simulink model "simulink_mecha_discrete_TEST"  (R2016b)
settings: Solver=ode1  StartTime=0.0  StopTime=10  FixedStep=0.01  RelTol=1e-6
undefined symbols (not defined in the file or in its folder): DiscIntNeverNeededParam
libraries: simulink x2, dspinverses x1
settings Model: Creator=Utente  LastModifiedBy=liana
settings DataIOCC: SaveState=on
settings OptimizationCC: BlockReduction=off  DefaultParameterBehavior=Inlined  BufferReuse=off

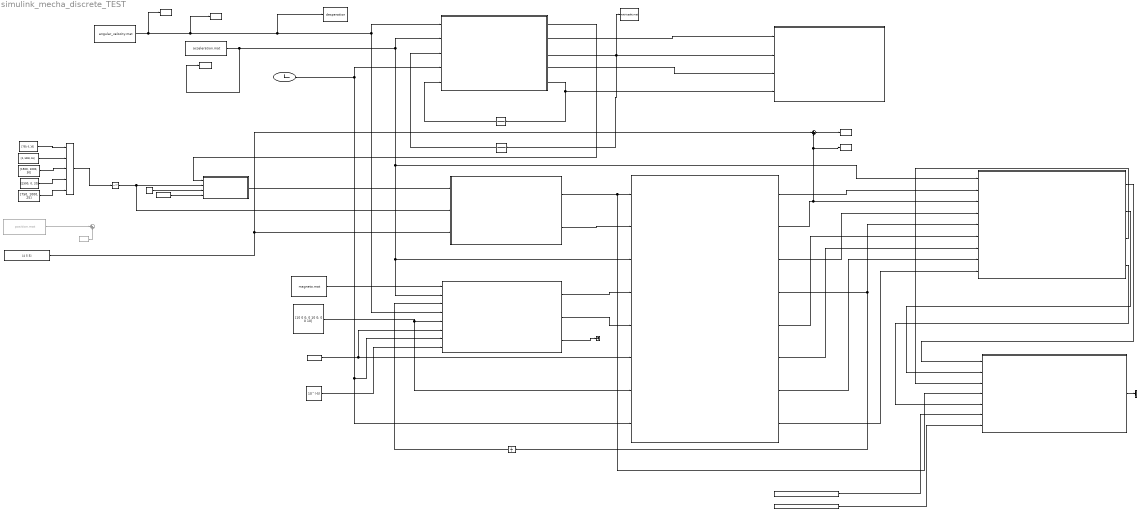
== system simulink_mecha_discrete_TEST ==
  Attitude Observer : Subsystem
  Band-Limited White Noise1 : simulink/Sources/Band-Limited White Noise  Commented=on  Cov=[0.1; 0.1; 0.1]  Ts=0.1  seed=[23341]
  Clock : Clock
      settings: Decimation=50
  Discrete-Time Integrator : DiscreteIntegrator  IntegratorMethod=Integration: Trapezoidal  InitialConditionSetting=State (most efficient)  SampleTime=-1  ICPrevOutput=DiscIntNeverNeededParam  ICPrevScaledInput=DiscIntNeverNeededParam
  Discrete-Time Integrator1 : DiscreteIntegrator  IntegratorMethod=Integration: Trapezoidal  InitialConditionSetting=State (most efficient)  SampleTime=-1  ICPrevOutput=DiscIntNeverNeededParam  ICPrevScaledInput=DiscIntNeverNeededParam
  Displays : Subsystem
  From  p_n_vehicle : FromFile  Commented=on  FileName=position.mat  SampleTime=0
  From acceleration file : FromFile  FileName=acceleration.mat  SampleTime=0
  From angular_velocity file : FromFile  FileName=angular_velocity.mat  SampleTime=0
  From magnetometer file : FromFile  FileName=magneto.mat  SampleTime=0  InterpolationWithinTimeRange=Zero order hold
  Kalman - Bucy Filter : Subsystem
  Kp : Constant  Value=[10 0 0; 0 10 0; 0 0 10]
  Local linearization1 : Subsystem
  Math Function : Math  Operator=transpose  SaturateOnIntegerOverflow=on
  Matrix Concatenate : Concatenate  NumInputs=5  Mode=Multidimensional array  ConcatenateDimension=2
  Mechanisation subsystem : Subsystem
  Nonlinear algebraic transform and solution : Subsystem
  Q matrix : Constant  Value=diag([0, 0, 0, 10^-5, 10^-3, 10^-3, 10^-3, 10^-8, 10^-8, 10^-8])
  R matrix : Constant  Value=0.25*diag([1 1 1 1])
  Sum : Sum  Inputs=|++
  Sum1 : Sum  Commented=on  Inputs=|++
  Terminator : Terminator
  Terminator2 : Terminator
  To File : ToFile  Filename=matricedot.mat  MatrixName=md  SaveFormat=Timeseries
  To Workspace : ToWorkspace  VariableName=desperation  SampleTime=-1
  To Workspace1 : ToWorkspace  VariableName=ang_vel  SampleTime=-1
  To Workspace2 : ToWorkspace  VariableName=ang_vel_dist  SampleTime=-1
  To Workspace3 : ToWorkspace  VariableName=accel  SaveFormat=Timeseries  SampleTime=-1
  To Workspace4 : ToWorkspace  VariableName=p_n  SaveFormat=Timeseries  SampleTime=-1
  To Workspace5 : ToWorkspace  VariableName=p_n_delta_stim  SaveFormat=Timeseries  SampleTime=-1
  Translational Motion Observer : Subsystem
  Unit Delay : UnitDelay  SampleTime=-1
  beta : Constant
  epsilon : Constant  Value=[1 1 1 1 1]
  ki : Constant  Value=10^(-5)
  p_n_1 : Constant  Value=[750, 0, 10]
  p_n_2 : Constant  Value=[0, 1000, 15]
  p_n_3 : Constant  Value=[1500, 1000, 30]
  p_n_4 : Constant  Value=[1500, 0, 20]
  p_n_5 : Constant  Value=[750, 1000, 25]
  position_0_fixed_reference : Constant  Value=[4 5 5]
  pseudorange_measurement_model : MATLAB Function  TreatAsAtomicUnit=on
  sigma : Constant  Value=0.25
  wires:
  Clock/1 -> Attitude Observer/7(t), Translational Motion Observer/8(t), Mechanisation subsystem/4(t)
  Mechanisation subsystem/3(R_nb_dot) -> Discrete-Time Integrator1/1, To File/1, Displays/2(R_nb_dot)
  Mechanisation subsystem/2(v_n_dot) -> Displays/1(v_n_dot)
  Mechanisation subsystem/4(v_n_dot_noise) -> Displays/3(v_n_dot_noise)
  Mechanisation subsystem/5(R_nb_dot_noise) -> Discrete-Time Integrator/1, Displays/4(R_nb_dot_noise)
  Discrete-Time Integrator/1 -> Mechanisation subsystem/5(R_nb_noise)
  Discrete-Time Integrator1/1 -> Mechanisation subsystem/3(R_nb)
  Nonlinear algebraic transform and solution/1(delta) -> Kalman - Bucy Filter/4(sensors measurements), Translational Motion Observer/1(delta)
  Translational Motion Observer/4(f_n_stim) -> Local linearization1/5(f_n_stim), Unit Delay/1
  Attitude Observer/1(J) -> Translational Motion Observer/4(J)
  Attitude Observer/2(R_nb_stim) -> Translational Motion Observer/5(R_nb_stim)
  Attitude Observer/3(b_stim) -> Terminator/1
  Kp/1 -> Translational Motion Observer/7(Kp), Attitude Observer/5(Kp)
  sigma/1 -> Attitude Observer/6(sigma), Translational Motion Observer/6(sigma)
  Translational Motion Observer/3(v_n_stim) -> Local linearization1/4(v_n_stim)
  Nonlinear algebraic transform and solution/2(C_dx) -> Translational Motion Observer/2(C_dx)
  Local linearization1/1(AL) -> Kalman - Bucy Filter/1(AL)
  Local linearization1/2(BL) -> Kalman - Bucy Filter/2(BL)
  Local linearization1/3(CL) -> Kalman - Bucy Filter/3(CL)
  pseudorange_measurement_model/1(y) -> Nonlinear algebraic transform and solution/1(y)
  Local linearization1/4(U) -> Kalman - Bucy Filter/5(U)
  beta/1 -> pseudorange_measurement_model/3(beta)
  epsilon/1 -> pseudorange_measurement_model/4(epsilon)
  Matrix Concatenate/1 -> Math Function/1
  R matrix/1 -> Kalman - Bucy Filter/6(R)
  Q matrix/1 -> Kalman - Bucy Filter/7(Q)
  Kalman - Bucy Filter/1(Out1) -> Terminator2/1
  Translational Motion Observer/5(K) -> Local linearization1/6(K)
  Translational Motion Observer/6("C ") -> Local linearization1/7(C)
  Translational Motion Observer/7(" A") -> Local linearization1/8(A)
  Translational Motion Observer/8(B) -> Local linearization1/9(B)
  ki/1 -> Attitude Observer/8(Ki)
  Unit Delay/1 -> Attitude Observer/3(f_n_stim)
  Band-Limited White Noise1/1 -> Sum1/2
  From  p_n_vehicle/1 -> Sum1/1
  Translational Motion Observer/1(beta_stim) -> Local linearization1/2(beta_stim)
  Translational Motion Observer/2(p_n_delta_stim) -> To Workspace5/1, Sum/2, Local linearization1/3(p_n_stim)
  Mechanisation subsystem/1(p_n) -> pseudorange_measurement_model/1(p_n)
  p_n_5/1 -> Matrix Concatenate/5
  p_n_4/1 -> Matrix Concatenate/4
  p_n_3/1 -> Matrix Concatenate/3
  p_n_2/1 -> Matrix Concatenate/2
  p_n_1/1 -> Matrix Concatenate/1
  Math Function/1 -> Nonlinear algebraic transform and solution/2(p), pseudorange_measurement_model/2(p_n_i)
  From angular_velocity file/1 -> To Workspace/1, Attitude Observer/4(w_ib), Mechanisation subsystem/1(w_ib), To Workspace2/1, To Workspace1/1
  From acceleration file/1 -> Local linearization1/1(f_b_imu), Attitude Observer/2(f_b), Translational Motion Observer/3(f_b_imu), Mechanisation subsystem/2(f_b), To Workspace3/1
  From magnetometer file/1 -> Attitude Observer/1(m_b_mag)
  Sum/1 -> To Workspace4/1
  position_0_fixed_reference/1 -> Sum/1, Nonlinear algebraic transform and solution/3(p0)

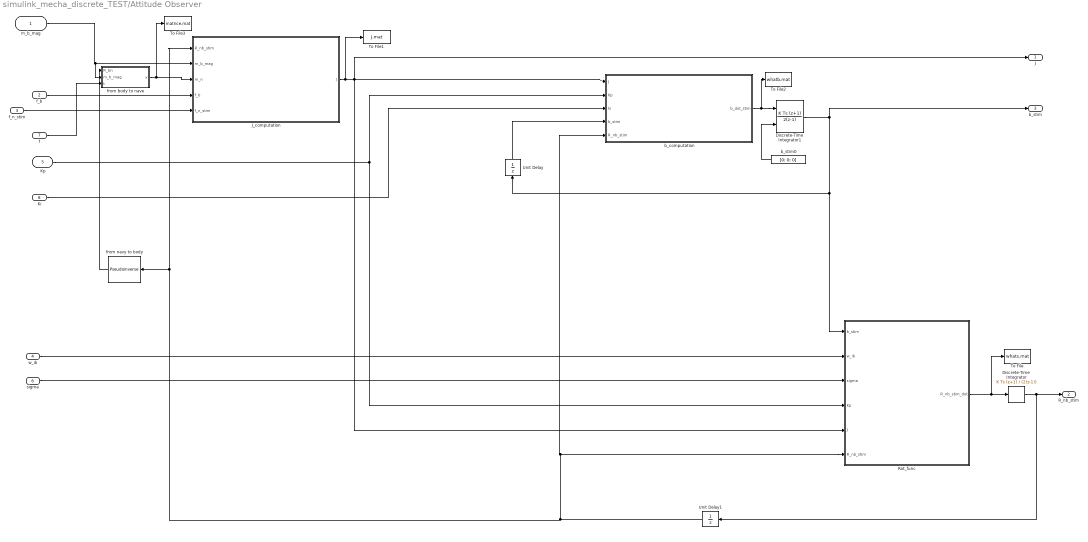
== system simulink_mecha_discrete_TEST/Attitude Observer ==
  m_b_mag : Inport
  f_b : Inport  Port=2
  f_n_stim : Inport  Port=3
  w_ib : Inport  Port=4
  Kp : Inport  Port=5
  sigma : Inport  Port=6
  t : Inport  Port=7
  Ki : Inport  Port=8
  Discrete-Time Integrator : DiscreteIntegrator  IntegratorMethod=Integration: Trapezoidal  InitialConditionSetting=State (most efficient)  SampleTime=-1  ICPrevOutput=DiscIntNeverNeededParam  ICPrevScaledInput=DiscIntNeverNeededParam
  Discrete-Time Integrator1 : DiscreteIntegrator  IntegratorMethod=Integration: Trapezoidal  InitialConditionSource=external  InitialConditionSetting=State (most efficient)  SampleTime=-1  ICPrevOutput=DiscIntNeverNeededParam  ICPrevScaledInput=DiscIntNeverNeededParam
  J_computation : Subsystem
  Rot_func : MATLAB Function  TreatAsAtomicUnit=on
  To File : ToFile  Filename=whats.mat  SaveFormat=Timeseries
  To File1 : ToFile  Filename=J.mat  MatrixName=J  SaveFormat=Timeseries
  To File2 : ToFile  Filename=whatb.mat  MatrixName=b  SaveFormat=Timeseries
  To File3 : ToFile  Filename=matrice.mat  MatrixName=m  SaveFormat=Timeseries
  Unit Delay : UnitDelay  SampleTime=-1
  Unit Delay1 : UnitDelay  SampleTime=-1
  b_computation : MATLAB Function  TreatAsAtomicUnit=on
  b_stim0 : Constant  Value=[0; 0; 0]
  from body to nave : MATLAB Function  TreatAsAtomicUnit=on
  from navy to body : dspinverses/Pseudoinverse  wanterr=off  SimulateUsing=Interpreted execution
  J : Outport
  R_nb_stim : Outport  Port=2
  b_stim : Outport  Port=3
  wires:
  m_b_mag/1 -> from body to nave/2(m_b_mag), J_computation/2(m_b_mag)
  Rot_func/1(R_nb_stim_dot) -> Discrete-Time Integrator/1, To File/1
  b_computation/1(b_dot_stim) -> Discrete-Time Integrator1/1, To File2/1
  Discrete-Time Integrator1/1 -> b_stim/1, Unit Delay/1, Rot_func/1(b_stim)
  from body to nave/1(y) -> J_computation/3(m_n), To File3/1
  f_b/1 -> J_computation/4(f_b)
  f_n_stim/1 -> J_computation/5(f_n_stim)
  J_computation/1(J) -> To File1/1, J/1, Rot_func/5(J), b_computation/1(J)
  Kp/1 -> b_computation/2(Kp), Rot_func/4(Kp)
  Ki/1 -> b_computation/3(ki)
  sigma/1 -> Rot_func/3(sigma)
  w_ib/1 -> Rot_func/2(w_ib)
  t/1 -> from body to nave/3(t)
  Discrete-Time Integrator/1 -> R_nb_stim/1, Unit Delay1/1
  Unit Delay/1 -> b_computation/4(b_stim)
  Unit Delay1/1 -> from navy to body/1, J_computation/1(R_nb_stim), b_computation/5(R_nb_stim), Rot_func/6(R_nb_stim)
  from navy to body/1 -> from body to nave/1(R_bn)
  b_stim0/1 -> Discrete-Time Integrator1/2

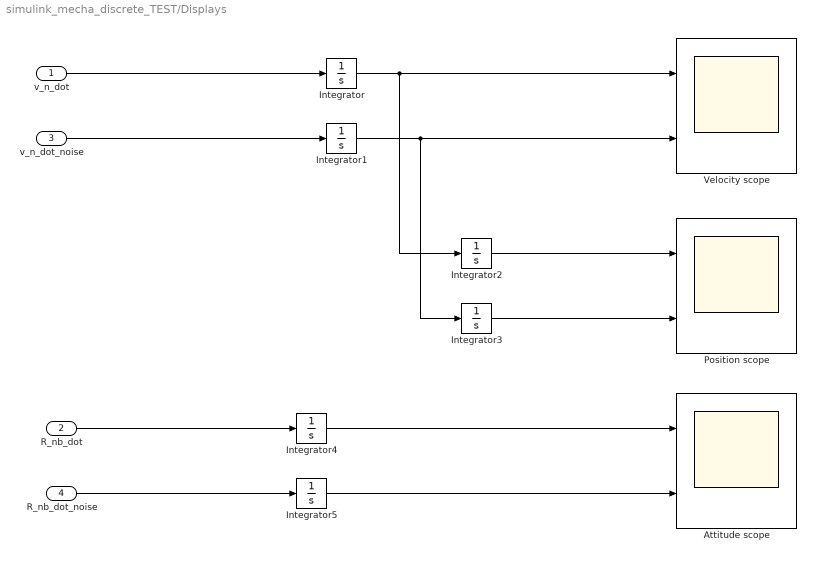
== system simulink_mecha_discrete_TEST/Displays ==
  v_n_dot : Inport
  R_nb_dot : Inport  Port=2
  v_n_dot_noise : Inport  Port=3
  R_nb_dot_noise : Inport  Port=4
  Attitude scope : Scope  NumInputPorts=2
  Integrator{,1..5} (6 alike) : Integrator
  Position scope : Scope  NumInputPorts=2
  Velocity scope : Scope  NumInputPorts=2
  wires:
  v_n_dot/1 -> Integrator/1
  v_n_dot_noise/1 -> Integrator1/1
  Integrator/1 -> Integrator2/1, Velocity scope/1
  Integrator1/1 -> Integrator3/1, Velocity scope/2
  Integrator2/1 -> Position scope/1
  Integrator3/1 -> Position scope/2
  R_nb_dot/1 -> Integrator4/1
  R_nb_dot_noise/1 -> Integrator5/1
  Integrator4/1 -> Attitude scope/1
  Integrator5/1 -> Attitude scope/2

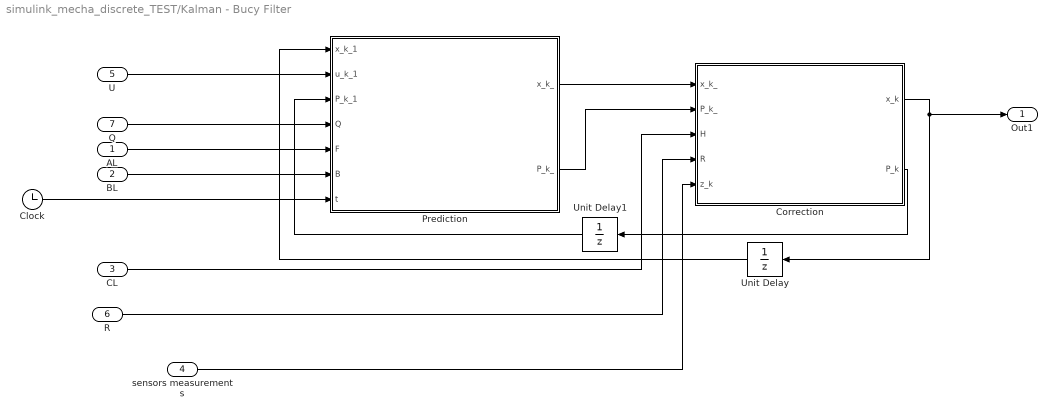
== system simulink_mecha_discrete_TEST/Kalman - Bucy Filter ==
  AL : Inport
  BL : Inport  Port=2
  CL : Inport  Port=3
  sensors measurements : Inport  Port=4
  U : Inport  Port=5
  R : Inport  Port=6
  Q : Inport  Port=7
  Clock : Clock
  Correction : MATLAB Function  TreatAsAtomicUnit=on
  Prediction : MATLAB Function  TreatAsAtomicUnit=on
  Unit Delay : UnitDelay  SampleTime=-1
  Unit Delay1 : UnitDelay  SampleTime=-1
  Out1 : Outport
  wires:
  Prediction/2(P_k_) -> Correction/2(P_k_)
  Prediction/1(x_k_) -> Correction/1(x_k_)
  Correction/2(P_k) -> Unit Delay1/1
  Correction/1(x_k) -> Unit Delay/1, Out1/1
  AL/1 -> Prediction/5(F)
  CL/1 -> Correction/3(H)
  Clock/1 -> Prediction/7(t)
  Q/1 -> Prediction/4(Q)
  sensors measurements/1 -> Correction/5(z_k)
  BL/1 -> Prediction/6(B)
  U/1 -> Prediction/2(u_k_1)
  R/1 -> Correction/4(R)
  Unit Delay/1 -> Prediction/1(x_k_1)
  Unit Delay1/1 -> Prediction/3(P_k_1)

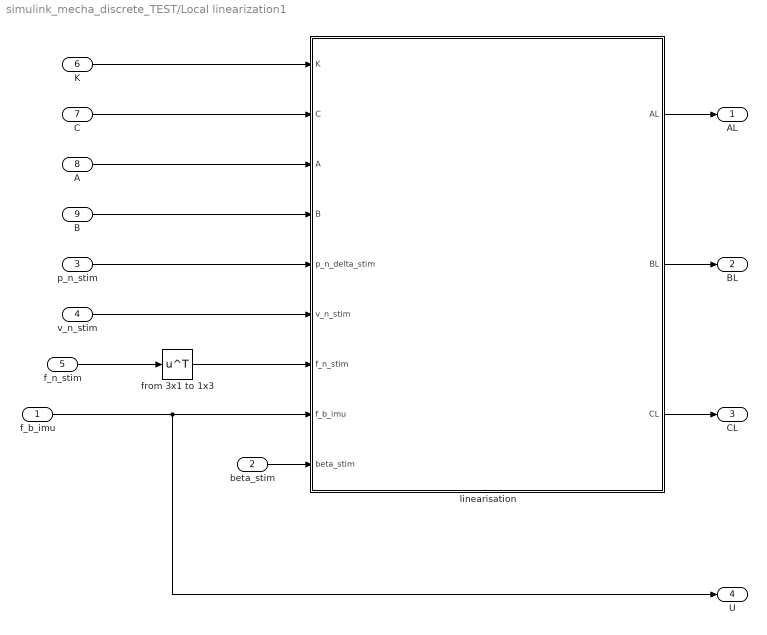
== system simulink_mecha_discrete_TEST/Local linearization1 ==
  f_b_imu : Inport
  beta_stim : Inport  Port=2
  p_n_stim : Inport  Port=3
  v_n_stim : Inport  Port=4
  f_n_stim : Inport  Port=5
  K : Inport  Port=6
  C : Inport  Port=7
  A : Inport  Port=8
  B : Inport  Port=9
  from 3x1 to 1x3 : Math  Operator=transpose  SaturateOnIntegerOverflow=on
  linearisation : MATLAB Function  TreatAsAtomicUnit=on
  AL : Outport
  BL : Outport  Port=2
  CL : Outport  Port=3
  U : Outport  Port=4
  wires:
  linearisation/1(AL) -> AL/1
  linearisation/2(BL) -> BL/1
  linearisation/3(CL) -> CL/1
  K/1 -> linearisation/1(K)
  C/1 -> linearisation/2(C)
  A/1 -> linearisation/3(A)
  B/1 -> linearisation/4(B)
  p_n_stim/1 -> linearisation/5(p_n_delta_stim)
  beta_stim/1 -> linearisation/9(beta_stim)
  f_n_stim/1 -> from 3x1 to 1x3/1
  v_n_stim/1 -> linearisation/6(v_n_stim)
  f_b_imu/1 -> U/1, linearisation/8(f_b_imu)
  from 3x1 to 1x3/1 -> linearisation/7(f_n_stim)

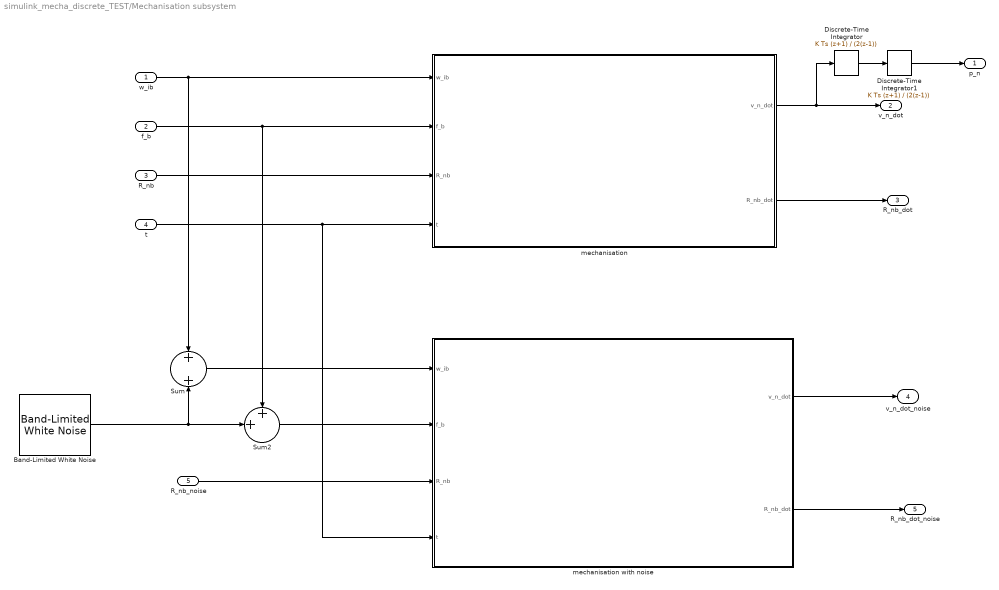
== system simulink_mecha_discrete_TEST/Mechanisation subsystem ==
  w_ib : Inport
  f_b : Inport  Port=2
  R_nb : Inport  Port=3
  t : Inport  Port=4
  R_nb_noise : Inport  Port=5
  Band-Limited White Noise : simulink/Sources/Band-Limited White Noise  Cov=[100 100 100]'  Ts=0.1  seed=[23341]  VectorParams1D=off
  Discrete-Time Integrator : DiscreteIntegrator  IntegratorMethod=Integration: Trapezoidal  InitialConditionSetting=State (most efficient)  SampleTime=-1  ICPrevOutput=DiscIntNeverNeededParam  ICPrevScaledInput=DiscIntNeverNeededParam
  Discrete-Time Integrator1 : DiscreteIntegrator  IntegratorMethod=Integration: Trapezoidal  InitialConditionSetting=State (most efficient)  SampleTime=-1  ICPrevOutput=DiscIntNeverNeededParam  ICPrevScaledInput=DiscIntNeverNeededParam
  Sum : Sum  Inputs=+|+
  Sum2 : Sum  Inputs=++|
  mechanisation : MATLAB Function  TreatAsAtomicUnit=on
  mechanisation with noise : MATLAB Function  TreatAsAtomicUnit=on
  p_n : Outport
  v_n_dot : Outport  Port=2
  R_nb_dot : Outport  Port=3
  v_n_dot_noise : Outport  Port=4
  R_nb_dot_noise : Outport  Port=5
  wires:
  w_ib/1 -> mechanisation/1(w_ib), Sum/1
  t/1 -> mechanisation with noise/4(t), mechanisation/4(t)
  R_nb/1 -> mechanisation/3(R_nb)
  f_b/1 -> Sum2/1, mechanisation/2(f_b)
  mechanisation/1(v_n_dot) -> Discrete-Time Integrator/1, v_n_dot/1
  mechanisation/2(R_nb_dot) -> R_nb_dot/1
  Band-Limited White Noise/1 -> Sum/2, Sum2/2
  Sum/1 -> mechanisation with noise/1(w_ib)
  Sum2/1 -> mechanisation with noise/2(f_b)
  mechanisation with noise/1(v_n_dot) -> v_n_dot_noise/1
  mechanisation with noise/2(R_nb_dot) -> R_nb_dot_noise/1
  R_nb_noise/1 -> mechanisation with noise/3(R_nb)
  Discrete-Time Integrator/1 -> Discrete-Time Integrator1/1
  Discrete-Time Integrator1/1 -> p_n/1

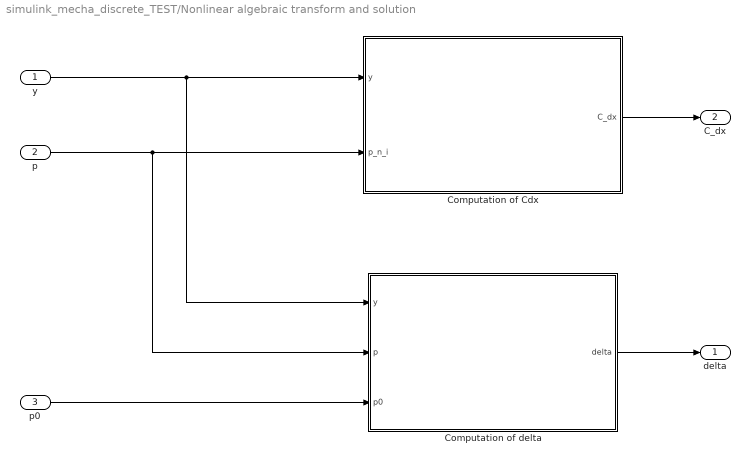
== system simulink_mecha_discrete_TEST/Nonlinear algebraic transform and solution ==
  y : Inport
  p : Inport  Port=2
  p0 : Inport  Port=3
  Computation of Cdx : MATLAB Function  TreatAsAtomicUnit=on
  Computation of delta : MATLAB Function  TreatAsAtomicUnit=on
  delta : Outport
  C_dx : Outport  Port=2
  wires:
  y/1 -> Computation of delta/1(y), Computation of Cdx/1(y)
  p/1 -> Computation of delta/2(p), Computation of Cdx/2(p_n_i)
  p0/1 -> Computation of delta/3(p0)
  Computation of delta/1(delta) -> delta/1
  Computation of Cdx/1(C_dx) -> C_dx/1

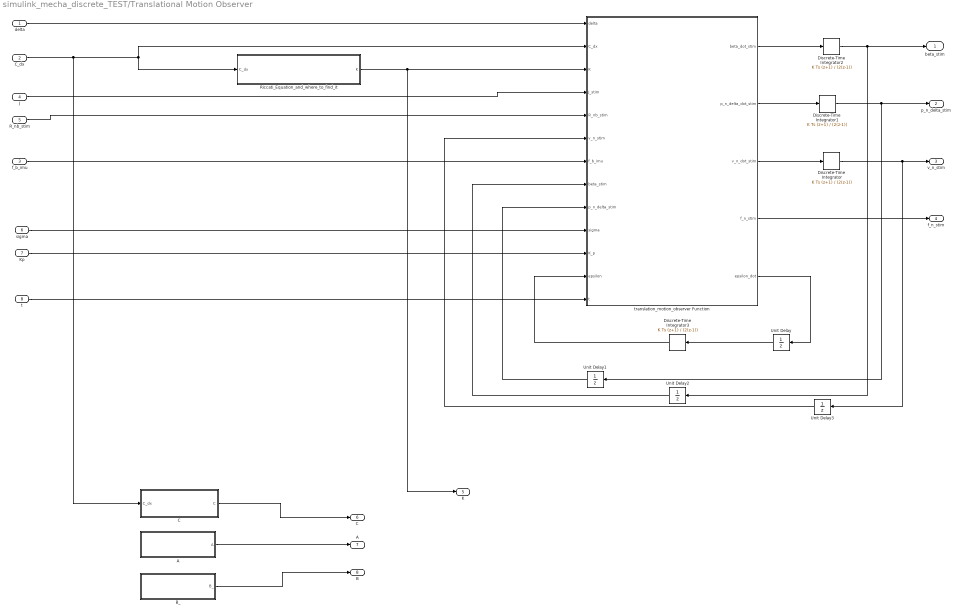
== system simulink_mecha_discrete_TEST/Translational Motion Observer ==
  delta : Inport
  C_dx : Inport  Port=2
  f_b_imu : Inport  Port=3
  J : Inport  Port=4
  R_nb_stim : Inport  Port=5
  sigma : Inport  Port=6
  Kp : Inport  Port=7
  t : Inport  Port=8
  A : MATLAB Function  TreatAsAtomicUnit=on
  B_ : MATLAB Function  TreatAsAtomicUnit=on
  C : MATLAB Function  TreatAsAtomicUnit=on
  Discrete-Time Integrator{,1..3} (4 alike) : DiscreteIntegrator  IntegratorMethod=Integration: Trapezoidal  InitialConditionSetting=State (most efficient)  SampleTime=-1  ICPrevOutput=DiscIntNeverNeededParam  ICPrevScaledInput=DiscIntNeverNeededParam
  Riccati_Equation_and_where_to_find_it : Subsystem
  Unit Delay{,1..3} (4 alike) : UnitDelay  SampleTime=-1
  translation_motion_observer Function : MATLAB Function  TreatAsAtomicUnit=on
  beta_stim : Outport
  p_n_delta_stim : Outport  Port=2
  v_n_stim : Outport  Port=3
  f_n_stim : Outport  Port=4
  K : Outport  Port=5
  "C " : Outport  Port=6
  " A" : Outport  Port=7
  B : Outport  Port=8
  wires:
  translation_motion_observer Function/4(f_n_stim) -> f_n_stim/1
  translation_motion_observer Function/3(v_n_dot_stim) -> Discrete-Time Integrator/1
  Discrete-Time Integrator/1 -> Unit Delay3/1, v_n_stim/1
  translation_motion_observer Function/2(p_n_delta_dot_stim) -> Discrete-Time Integrator1/1
  Discrete-Time Integrator1/1 -> p_n_delta_stim/1, Unit Delay1/1
  Discrete-Time Integrator2/1 -> beta_stim/1, Unit Delay2/1
  translation_motion_observer Function/1(beta_dot_stim) -> Discrete-Time Integrator2/1
  translation_motion_observer Function/5(epsilon_dot) -> Unit Delay/1
  C_dx/1 -> C/1(C_dx), Riccati_Equation_and_where_to_find_it/1(C_dx), translation_motion_observer Function/2(C_dx)
  J/1 -> translation_motion_observer Function/4(J_stim)
  R_nb_stim/1 -> translation_motion_observer Function/5(R_nb_stim)
  delta/1 -> translation_motion_observer Function/1(delta)
  f_b_imu/1 -> translation_motion_observer Function/7(f_b_imu)
  sigma/1 -> translation_motion_observer Function/10(sigma)
  Kp/1 -> translation_motion_observer Function/11(K_p)
  A/1(A) -> " A"/1
  C/1(C) -> "C "/1
  Riccati_Equation_and_where_to_find_it/1(K) -> K/1, translation_motion_observer Function/3(K)
  B_/1(B_) -> B/1
  t/1 -> translation_motion_observer Function/13(t)
  Discrete-Time Integrator3/1 -> translation_motion_observer Function/12(epsilon)
  Unit Delay1/1 -> translation_motion_observer Function/9(p_n_delta_stim)
  Unit Delay2/1 -> translation_motion_observer Function/8(beta_stim)
  Unit Delay3/1 -> translation_motion_observer Function/6(v_n_stim)
  Unit Delay/1 -> Discrete-Time Integrator3/1

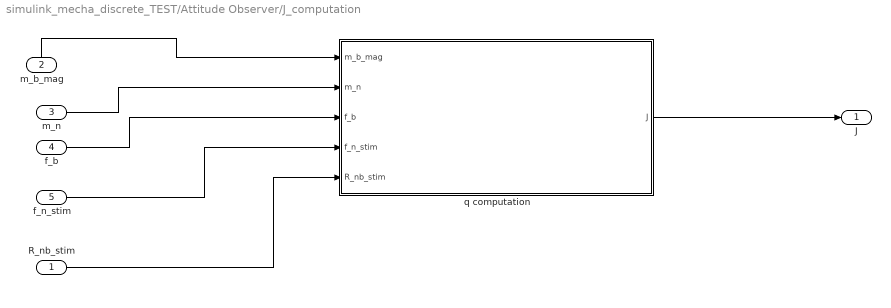
== system simulink_mecha_discrete_TEST/Attitude Observer/J_computation ==
  R_nb_stim : Inport
  m_b_mag : Inport  Port=2
  m_n : Inport  Port=3
  f_b : Inport  Port=4
  f_n_stim : Inport  Port=5
  q computation : MATLAB Function  TreatAsAtomicUnit=on
  J : Outport
  wires:
  m_n/1 -> q computation/2(m_n)
  f_n_stim/1 -> q computation/4(f_n_stim)
  m_b_mag/1 -> q computation/1(m_b_mag)
  f_b/1 -> q computation/3(f_b)
  q computation/1(J) -> J/1
  R_nb_stim/1 -> q computation/5(R_nb_stim)

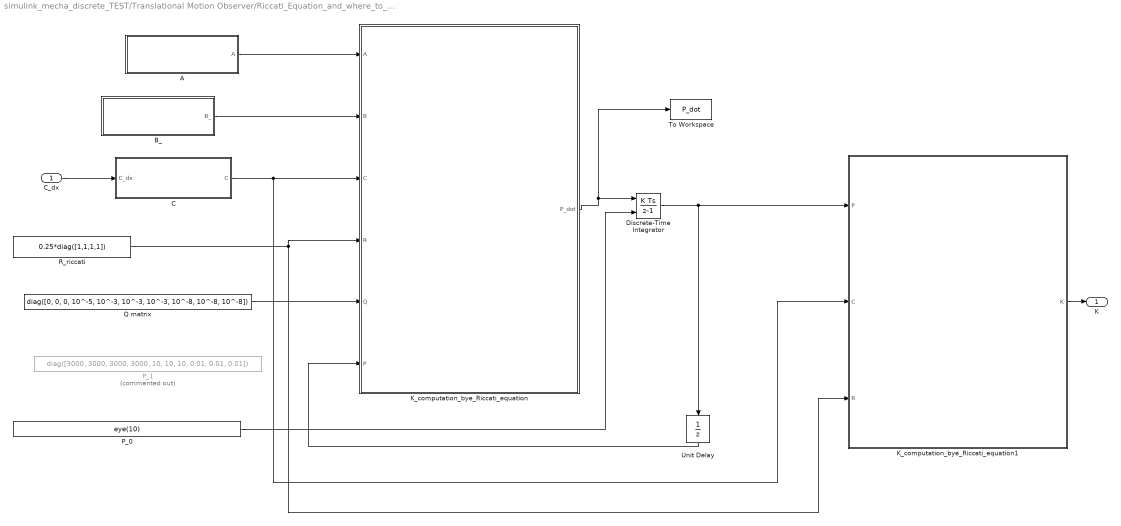
== system simulink_mecha_discrete_TEST/Translational Motion Observer/Riccati_Equation_and_where_to_find_it ==
  C_dx : Inport
  A : MATLAB Function  TreatAsAtomicUnit=on
  B_ : MATLAB Function  TreatAsAtomicUnit=on
  C : MATLAB Function  TreatAsAtomicUnit=on
  Discrete-Time Integrator : DiscreteIntegrator  InitialConditionSource=external  InitialConditionSetting=State (most efficient)  SampleTime=-1  ICPrevOutput=DiscIntNeverNeededParam  ICPrevScaledInput=DiscIntNeverNeededParam
  K_computation_bye_Riccati_equation : MATLAB Function  TreatAsAtomicUnit=on
  K_computation_bye_Riccati_equation1 : MATLAB Function  TreatAsAtomicUnit=on
  P_0 : Constant  Value=eye(10)
  P_1 : Constant  Commented=on  Value=diag([3000, 3000, 3000, 3000, 10, 10, 10, 0.01, 0.01, 0.01])
  Q matrix : Constant  Value=diag([0, 0, 0, 10^-5, 10^-3, 10^-3, 10^-3, 10^-8, 10^-8, 10^-8])
  R_riccati : Constant  Value=0.25*diag([1,1,1,1])
  To Workspace : ToWorkspace  VariableName=P_dot  SampleTime=-1
  Unit Delay : UnitDelay  SampleTime=-1
  K : Outport
  wires:
  C_dx/1 -> C/1(C_dx)
  R_riccati/1 -> K_computation_bye_Riccati_equation/4(R), K_computation_bye_Riccati_equation1/3(R)
  A/1(A) -> K_computation_bye_Riccati_equation/1(A)
  Q matrix/1 -> K_computation_bye_Riccati_equation/5(Q)
  C/1(C) -> K_computation_bye_Riccati_equation/3(C), K_computation_bye_Riccati_equation1/2(C)
  B_/1(B_) -> K_computation_bye_Riccati_equation/2(B)
  K_computation_bye_Riccati_equation1/1(K) -> K/1
  K_computation_bye_Riccati_equation/1(P_dot) -> Discrete-Time Integrator/1, To Workspace/1
  Discrete-Time Integrator/1 -> Unit Delay/1, K_computation_bye_Riccati_equation1/1(P)
  Unit Delay/1 -> K_computation_bye_Riccati_equation/6(P)
  P_0/1 -> Discrete-Time Integrator/2

== matlab function simulink_mecha_discrete_TEST/Translational Motion Observer/Riccati_Equation_and_where_to_find_it/B_ ==
  data: B_ output
function B_ = B()

 B_ = zeros(10,3);

 B_(8:10,1:3) = eye(3);
end

== matlab function simulink_mecha_discrete_TEST/Attitude Observer/J_computation/q computation ==
  data: m_b_mag input; m_n input; f_b input; f_n_stim input size=3; J output; R_nb_stim input size=[3,3]
function J  = qEfunc(m_b_mag, m_n, f_b, f_n_stim, R_nb_stim)

g_n = [0 0 9.81]';

q1_b = m_b_mag/norm(m_b_mag,2);
q2_b = f_b/norm(g_n,2);

q1_n = m_n/norm(m_n,2);
q2_n = f_n_stim/norm(g_n,2);


E_b = [q1_b, skew(q1_b)*q2_b, (skew(q1_b)*skew(q1_b))*q2_b];
E_n = [q1_n, skew(q1_n)*q2_n, (skew(q1_n)*skew(q1_n))*q2_n];

J = (E_n - R_nb_stim * E_b) * (E_b');

end

== matlab function simulink_mecha_discrete_TEST/Kalman - Bucy Filter/Prediction ==
  data: x_k_1 input size=[10, 1]; x_k_ output; u_k_1 input; P_k_1 input size=[10,10]; Q input; F input; B input; P_k_ output; t input
function [x_k_, P_k_] = prediction(x_k_1, u_k_1, P_k_1, Q, F,B, t)

    % initial value of x_k_1
    if t == 0
        x_k_1 = zeros(10,1);
    end

    x_k_ = F * x_k_1 + B * u_k_1;
    
    P_k_ = F * P_k_1 * F' + Q;
    

end

== matlab function simulink_mecha_discrete_TEST/Mechanisation subsystem/mechanisation ==
  data: w_ib input; f_b input; v_n_dot output; R_nb_dot output; R_nb input; t input
function [v_n_dot, R_nb_dot] = mechanisation(w_ib, f_b, R_nb, t)



g_n = [0 0 9.81]';

% w_ib = size(3,1);

if t == 0
    v_n_dot = ones(3,1);
    R_nb_dot = eye(3);
    R_nb = eye(3);
end

% mechanisation

% Skew = zeros(3,3);
% Skew(1,2) = -w_ib(3);
% Skew(2,1) = w_ib(3);
% Skew(1,3) = w_ib(2);
% Skew(3,1) = -w_ib(2);
% Skew(2,3) = -w_ib(1);
% Skew(3,2) = w_ib(1);

Skew = skew(w_ib);


%p_dot = v_n;
v_n_dot = R_nb * f_b + g_n;
R_nb_dot = R_nb * Skew;

== matlab function simulink_mecha_discrete_TEST/Mechanisation subsystem/mechanisation with noise ==
  data: w_ib input; f_b input; v_n_dot output; R_nb_dot output; R_nb input; t input
function [v_n_dot, R_nb_dot] = mechanisation(w_ib, f_b, R_nb, t)



g_n = [0 0 1]';

% w_ib = size(3,1);

if t == 0
    v_n_dot = zeros(3,1);
    R_nb_dot = eye(3);
    R_nb = eye(3);
end

% mechanisation

% Skew = zeros(3,3);
% Skew(1,2) = -w_ib(3);
% Skew(2,1) = w_ib(3);
% Skew(1,3) = w_ib(2);
% Skew(3,1) = -w_ib(2);
% Skew(2,3) = -w_ib(1);
% Skew(3,2) = w_ib(1);
Skew = skew(w_ib);


%p_dot = v_n;
v_n_dot = R_nb * f_b + g_n;
R_nb_dot = R_nb * Skew;

== matlab function simulink_mecha_discrete_TEST/Attitude Observer/b_computation ==
  data: J input; b_dot_stim output size=3; Kp input; ki input; b_stim input; R_nb_stim input
function b_dot_stim = b_dot_stim_func(J, Kp, ki, b_stim, R_nb_stim)

% don't break balls if there are too rows

%b_dot_stim = zeros(3 ,1);

% if t == 0
%    
%     b_stim = zeros(3, 1);
%     
% end

SAT = sat(R_nb_stim)';
PA = pa( SAT * Kp * J);
VEX = vexfunc(PA);
b_dot_stim = Proj(b_stim , -ki * VEX);

end

== matlab function simulink_mecha_discrete_TEST/Translational Motion Observer/translation_motion_observer Function ==
  data: delta input; C_dx input; K input; beta_dot_stim output; J_stim input; R_nb_stim input; p_n_delta_dot_stim output; v_n_dot_stim output; f_n_stim output size=[3,1]; v_n_stim input size=3; f_b_imu input size=3; beta_stim input; p_n_delta_stim input size=3; sigma input; K_p input; epsilon_dot output; epsilon input size=3; t input
function [beta_dot_stim,p_n_delta_dot_stim,v_n_dot_stim,f_n_stim,epsilon_dot] =  TMO_func(delta,C_dx,K,J_stim,R_nb_stim, v_n_stim,f_b_imu, beta_stim, p_n_delta_stim,sigma,K_p,epsilon,t)

 K_pp = K(1:3,:); 
 K_beta_p = K(4,:);
 K_v_p = K(5:7,:);
 K_eps_p = K(8:10,:);
 %obtained by Riccati equation..


% remember to insert a clock to define dimensions of all variables
g_n = [0 0 9.81]';

if(t == 0) 
   
    delta_stim = zeros(3, 1);
    delta_diff = zeros(3, 1);
    v_n_stim = zeros(3, 1);
    beta_stim = 0;
    epsilon = zeros(3,1);
    p_n_delta_stim = zeros(3, 1);
        
end



x_stim = [p_n_delta_stim; beta_stim];
%delta_stim = 2*C_dx*x_stim;
%delta_diff = (delta - delta_stim);



p_n_delta_dot_stim = v_n_stim + K_pp * (delta - 2*C_dx*x_stim);       % eq 14


beta_dot_stim = K_beta_p * (delta - 2*C_dx*x_stim);                       % eq 15


%theoretically we can't know epsilon
f_n_stim = R_nb_stim*f_b_imu + epsilon ;         % eq 18


v_n_dot_stim  = f_n_stim + g_n + K_v_p*(delta - 2*C_dx*x_stim);         % eq 16


epsilon_dot   = -sigma*K_p*J_stim*f_b_imu + K_eps_p*(delta - 2*C_dx*x_stim); % eq 17
end

== matlab function simulink_mecha_discrete_TEST/Nonlinear algebraic transform and solution/Computation of Cdx ==
  data: y input; p_n_i input; C_dx output size=[4,4]
function C_dx  = C_dx_func(y,p_n_i)

    % y vector 
    % p matrix has row vectors
    %            (x,y,z) cols 
    %            m-rows are transponders number
    % all variables are in navigation frame oh yeah! baby ;)
    
    [row,col] = size(p_n_i);
    [row_,col_] = size(y);
    
    % m-measure vector
    p_m = p_n_i(row,:);
    y_m = y(row_);

    m = row; % m is transpoders number
    
    
    p_ = zeros(m-1,3); %row vector, 3 stands for x,y,z
    y_ = zeros(m-1,1);
    
    for i = 1 : 1 : m-1
    
        p_(i,:) = p_m - p_n_i(i,:);
        y_(i) = y(i) - y_m;
        
    end
    
    C_dx = [p_, y_];

end

== matlab function simulink_mecha_discrete_TEST/Nonlinear algebraic transform and solution/Computation of delta ==
  data: y input; delta output size=4; p input; p0 input
function delta  = delta_func(y,p,p0)

    % y vector 
    % p matrix has row vectors
    %            (x,y,z) cols 
    %            m-rows are the numbers of the transponders
    % all variables are in navigation frame oh yeah! baby ;)
    % z is a col vector of scalars
    
    % we must choose p0 (a block)
    
    [row,col] = size(p);
    %[row_,col_] = size(y);
    
    p_los = zeros(row,col);
    z = zeros(row,1);
    %defining los vector
    
    for i = 1:1:row
       p_los(i,:) = p(i,:) - p0';
    end
    
    % p_los = p_los';
    
    for i = 1:1:row
        z(i)= (y(i)^2-norm(p_los(i,:))^2);
    end
    
    z = z';
    
    delta = zeros(row-1,1);
    z_m = z(end);
    
    for i = 1:1:row-1
        delta(i) =  (z(i) - z_m); %amm fenito
    end
    
    delta;

end

== matlab function simulink_mecha_discrete_TEST/Translational Motion Observer/Riccati_Equation_and_where_to_find_it/K_computation_bye_Riccati_equation ==
  data: A input; B input; P_dot output; C input; R input; Q input; P input size=[10, 10]
function P_dot = P_dot_func(A,B,C,R,Q,P)

P_dot = P*A + A.'*P - P*C.'*(R\C)*P + Q;

end

== matlab function simulink_mecha_discrete_TEST/Translational Motion Observer/Riccati_Equation_and_where_to_find_it/A ==
  data: A output
function A = A()

 A = zeros(10);

 A(1:3,5:7) = eye(3);
 A(5:7,8:10) = eye(3);
 
end

== matlab function simulink_mecha_discrete_TEST/Translational Motion Observer/Riccati_Equation_and_where_to_find_it/C ==
  data: C output; C_dx input
function C = C(C_dx)

   row = size(C_dx,1); 

   C1 = zeros(row,6);

 C = [2*C_dx C1];

== matlab function simulink_mecha_discrete_TEST/Attitude Observer/Rot_func ==
  data: b_stim input; R_nb_stim_dot output; w_ib input; sigma input; Kp input; J input; R_nb_stim input
function R_nb_stim_dot = rot_func(b_stim,w_ib,sigma,Kp,J,R_nb_stim) 

Skew = skew(w_ib - b_stim);

R_nb_stim_dot = R_nb_stim * Skew + sigma * Kp * J;

== matlab function simulink_mecha_discrete_TEST/Kalman - Bucy Filter/Correction ==
  data: x_k_ input; P_k_ input size=[10,10]; H input; R input; z_k input; x_k output; P_k output
function [x_k, P_k] = correction(x_k_ ,P_k_, H, R, z_k)

    n = size(P_k_);


    K_k = P_k_ * H' * pinv(H * P_k_ * H' + R);
    
    x_k = x_k_ + K_k * (z_k - H * x_k_);
    
    P_k = (eye(n) - K_k * H)*P_k_;

end

== matlab function simulink_mecha_discrete_TEST/Translational Motion Observer/A ==
  data: A output
function A = A()

 A = zeros(10);

 A(1:3,5:7) = eye(3);
 A(5:7,8:10) = eye(3);
 
end

== matlab function simulink_mecha_discrete_TEST/Translational Motion Observer/C ==
  data: C output; C_dx input
function C = Cfunc(C_dx)

   row = size(C_dx,1); 

   C1 = zeros(row,6);

 C = [2*C_dx C1];
 
 
end

== matlab function simulink_mecha_discrete_TEST/Translational Motion Observer/B_ ==
  data: B_ output
function B_ = B()

 B_ = zeros(10,3);

 B_(8:10,1:3) = eye(3);
end

== matlab function simulink_mecha_discrete_TEST/pseudorange_measurement_model ==
  data: p_n input; y output size=5; p_n_i input; beta input; epsilon input
function y = pseudorange_mea_model(p_n,p_n_i,beta,epsilon)

  %  row-vector

  y = zeros(size(p_n_i,1),1);

  for i = 1: size(p_n_i,1)

      rho = norm(p_n-p_n_i(i,:)');  % eq. 7
      
      y(i) = rho + beta + epsilon(i); % eq. 8 

  end
      
end

== matlab function simulink_mecha_discrete_TEST/Translational Motion Observer/Riccati_Equation_and_where_to_find_it/K_computation_bye_Riccati_equation1 ==
  data: P input; K output; C input; R input
function K = K_func(P, C, R)

K = zeros(10,size(C,1));

R_inv = pinv(R);

K = P*C'*R_inv;

end

== matlab function simulink_mecha_discrete_TEST/Local linearization1/linearisation ==
  data: K input size=[10,4]; AL output size=[10,10]; BL output size=[10,3]; CL output size=[4,10]; C input size=[4,10]; A input size=[10,10]; B input size=[10,3]; p_n_delta_stim input size=[1,3]; v_n_stim input size=[1,3]; f_n_stim input size=[1,3]; f_b_imu input size=[1,3]; beta_stim input size=1
function [AL, BL, CL] = linearisation(K,C,A,B, p_n_delta_stim, v_n_stim, f_n_stim, f_b_imu, beta_stim)

 % building state vector
 % xsi = [p_n_stim ; beta_stim; v_n_stim; f_n_tim];
%   xsi = zeros(10,1);
%   xsi(1:3,1) = p_n_delta_stim;
%   xsi(4,1) = beta_stim;
%   xsi(5:7,1) = v_n_stim;
%   xsi(8:10,1) = f_n_stim;
 % coder.extrinsic('ss');
 % sys = ss(A-K*C,B,C,0);
% % getting work point
%coder.extrinsic('trim');
%[X,U,Y,DX] = trim('sys', xsi);

% computing linearisation model
%coder.extrinsic('linmod');
%[AL, BL, CL, DL] = linmod('sys',X,U);

  
AL = zeros(10,10);
BL = zeros(10,3);
CL = zeros(size(C,1), 10);


coder.extrinsic('LinearizationFun');

[Al,Bl,Cl] = LinearizationFun(K,C,A,B);

p_n0 = p_n_delta_stim(1, 1);
p_n1 = p_n_delta_stim (1,2);
p_n2 = p_n_delta_stim(1,3);

v_n0 = v_n_stim(1, 1);
v_n1 = v_n_stim(1,2);
v_n2 = v_n_stim(1,3);

f_n0 = f_n_stim(1,1);
f_n1 = f_n_stim(1,2);
f_n2 = f_n_stim(1,3);

f_b0 = f_b_imu(1,1);
f_b1 = f_b_imu(1,2);
f_b2 = f_b_imu(1,3);


coder.extrinsic('eval');

AL_ = eval(Al);
BL_ = eval(Bl);
CL_ = eval(Cl);

% AL_ = feval('Al', p_n0, p_n1, p_n2,v_n0, v_n1, v_n2, f_n0, f_n1, f_n2, beta_stim);
% BL_ = feval('Bl', f_b0, f_b1, f_b2);
% CL_ = feval('Cl', p_n0, p_n1, p_n2,v_n0, v_n1, v_n2, f_n0, f_n1, f_n2, beta_stim);
% 

AL = AL_;
BL = BL_;
CL = CL_;


end

== matlab function simulink_mecha_discrete_TEST/Attitude Observer/from body to nave ==
  data: R_bn input; y output; m_b_mag input; t input
function y = b2n(R_bn, m_b_mag,t)

if t==0
    R_bn = eye(3);
end

y = R_bn * m_b_mag;
